simulink model "ElectricVehicle"  (R2022b)
settings: Solver=VariableStepAuto  StartTime=0  StopTime=350  RelTol=1e-3
libraries: autolibshared x1, slpidlib x1
settings Model: Creator=frz  LastModifiedBy=frz
settings SolverCC: ZeroCrossAlgorithm=Adaptive
settings DataIOCC: SaveOutput=off  SaveTime=off  ReturnWorkspaceOutputs=off
settings DebuggingCC: MaskedZcDiagnostic=none  IgnoredZcDiagnostic=none

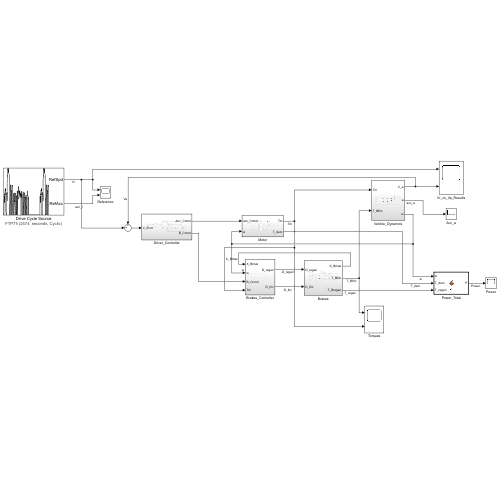
[thumbnail: Simulink's stored preview of the top-level diagram]
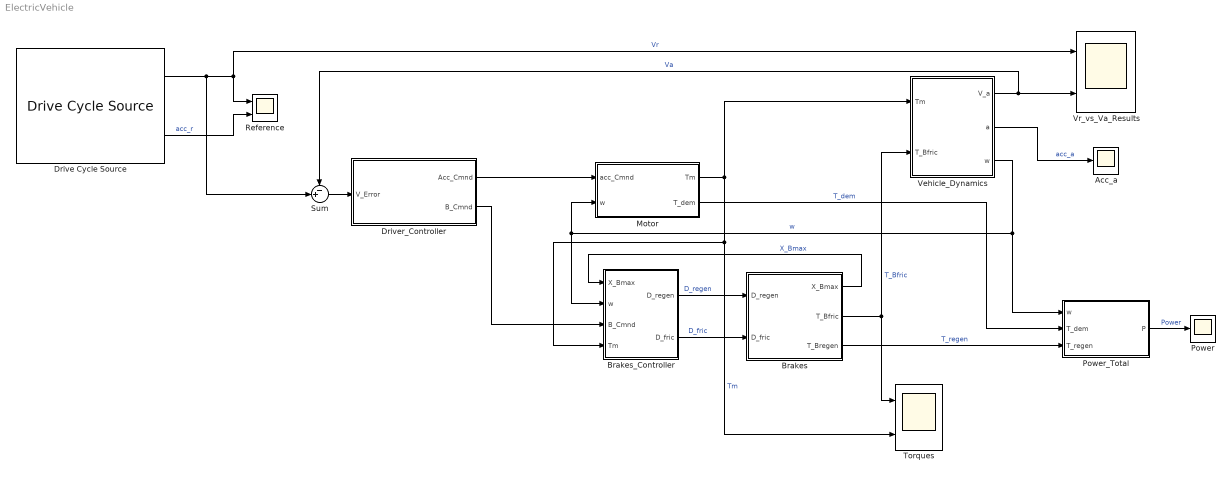
== system ElectricVehicle ==
  Acc_a : Scope
  Brakes : Subsystem
  Brakes_Controller : Subsystem
  Drive Cycle Source : autolibshared/Drive Cycle Source  cycleVar=FTP75  fileVar=cycleFTP75.mat  tfinal="2474  seconds, Cyclic"  cycleRepeat=on  outAccPort=on  outGearPort=off  gearList=No gear data  t_wot1=5  xdot_woto=0  xdot_wot1=30  t_wot2=20  xdot_wot2=0  t_wotend=30  srcUnit=m/s  outUnit=km/h  srcAccUnit=m/s/s  outAccUnit=m/s^2  dt=0  aMode=1  faultOption=off  velBnd=2  velBndUnit=mph  inUnit=m/s  timeBnd=1  failOption=off  stopSim=off  maxFaultCnt=10  maxFaultTime=2  maxTotFaultTime=15  traceOption=off  dtTrace=1  traceWindow=10  lastDCname=FTP75  lastOutUnit=mph  lastDT=0  lastTB=1  lastSB=2  forceCalcBound=off
  Driver_Controller : Subsystem
  Motor : Subsystem
  Power : Scope
  Power_Total : MATLAB Function  TreatAsAtomicUnit=on
  Reference : Scope  NumInputPorts=2
  Sum : Sum  Inputs=-+|
  Torques : Scope  NumInputPorts=2
  Vehicle_Dynamics : Subsystem
  Vr_vs_Va_Results : Scope  NumInputPorts=2
  wires:
  Drive Cycle Source/1 -> Sum/2, Reference/1, Vr_vs_Va_Results/1  "Vr"
  Drive Cycle Source/2 -> Reference/2  "acc_r"
  Brakes/2(T_Bfric) -> Vehicle_Dynamics/2(T_Bfric), Torques/1  "T_Bfric"
  Brakes/1(X_Bmax) -> Brakes_Controller/1(X_Bmax)  "X_Bmax"
  Brakes_Controller/1(D_regen) -> Brakes/1(D_regen)  "D_regen"
  Brakes_Controller/2(D_fric) -> Brakes/2(D_fric)  "D_fric"
  Brakes/3(T_Bregen) -> Power_Total/3(T_regen)  "T_regen"
  Vehicle_Dynamics/3(w) -> Power_Total/1(w), Motor/2(w), Brakes_Controller/2(w)  "w"
  Vehicle_Dynamics/1(V_a) -> Vr_vs_Va_Results/2, Sum/1  "Va"
  Driver_Controller/1(Acc_Cmnd) -> Motor/1(acc_Cmnd)
  Driver_Controller/2(B_Cmnd) -> Brakes_Controller/3(B_Cmnd)
  Sum/1 -> Driver_Controller/1(V_Error)
  Motor/1(Tm) -> Torques/2, Brakes_Controller/4(Tm), Vehicle_Dynamics/1(Tm)  "Tm"
  Vehicle_Dynamics/2(a) -> Acc_a/1  "acc_a"
  Motor/2(T_dem) -> Power_Total/2(T_dem)  "T_dem"
  Power_Total/1(P) -> Power/1  "Power"

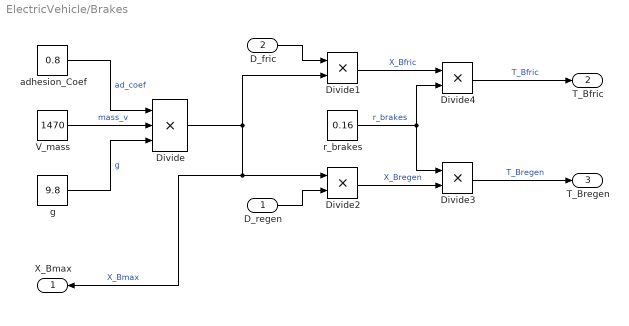
== system ElectricVehicle/Brakes ==
  D_regen : Inport
  D_fric : Inport  Port=2
  Divide : Product  Inputs=***
  Divide{1..4} (4 alike) : Product  Inputs=**
  V_mass : Constant  Value=1470
  adhesion_Coef : Constant  Value=0.8
  g : Constant  Value=9.8
  r_brakes : Constant  Value=0.16
  X_Bmax : Outport
  T_Bfric : Outport  Port=2
  T_Bregen : Outport  Port=3
  wires:
  g/1 -> Divide/3  "g"
  adhesion_Coef/1 -> Divide/1  "ad_coef"
  V_mass/1 -> Divide/2  "mass_v"
  D_fric/1 -> Divide1/1
  Divide1/1 -> Divide4/1  "X_Bfric"
  Divide4/1 -> T_Bfric/1  "T_Bfric"
  r_brakes/1 -> Divide3/1, Divide4/2  "r_brakes"
  D_regen/1 -> Divide2/2
  Divide/1 -> Divide1/2, X_Bmax/1, Divide2/1  "X_Bmax"
  Divide2/1 -> Divide3/2  "X_Bregen"
  Divide3/1 -> T_Bregen/1  "T_Bregen"

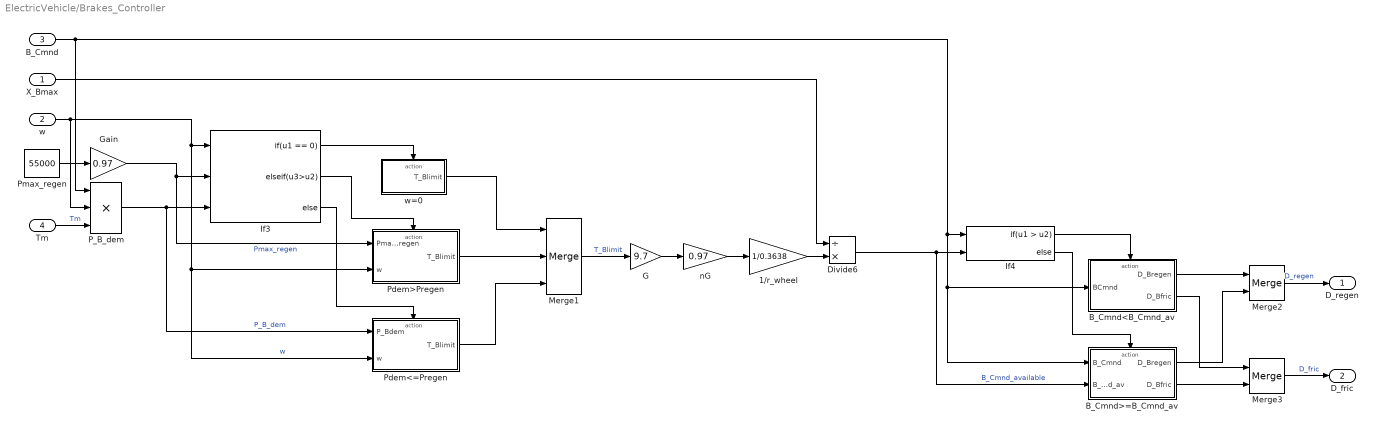
== system ElectricVehicle/Brakes_Controller ==
  X_Bmax : Inport
  w : Inport  Port=2
  B_Cmnd : Inport  Port=3
  Tm : Inport  Port=4
  1/r_wheel : Gain  Gain=1/0.3638
  B_Cmnd<B_Cmnd_av : Subsystem  TreatAsAtomicUnit=on
  B_Cmnd>=B_Cmnd_av : Subsystem  TreatAsAtomicUnit=on
  Divide6 : Product  Inputs=/*
  G : Gain  Gain=9.7
  Gain : Gain  Gain=0.97
  If3 : If  NumInputs=3  IfExpression=u1 == 0  ElseIfExpressions=u3>u2
  If4 : If  NumInputs=2  IfExpression=u1 > u2
  Merge1 : Merge  Inputs=3
  Merge2 : Merge
  Merge3 : Merge
  P_B_dem : Product  Inputs=***
  Pdem<=Pregen : Subsystem  TreatAsAtomicUnit=on
  Pdem>Pregen : Subsystem  TreatAsAtomicUnit=on
  Pmax_regen : Constant  Value=55000
  nG : Gain  Gain=0.97
  w=0 : Subsystem  TreatAsAtomicUnit=on
  D_regen : Outport
  D_fric : Outport  Port=2
  wires:
  Pdem<=Pregen/1(T_Blimit) -> Merge1/3
  If3/1 -> w=0/Action
  Pmax_regen/1 -> Gain/1
  B_Cmnd/1 -> If4/1, B_Cmnd<B_Cmnd_av/1(BCmnd), B_Cmnd>=B_Cmnd_av/1(B_Cmnd), P_B_dem/1
  X_Bmax/1 -> Divide6/1
  Merge2/1 -> D_regen/1  "D_regen"
  If3/2 -> Pdem>Pregen/Action
  P_B_dem/1 -> If3/3, Pdem<=Pregen/1(P_Bdem)  "P_B_dem"
  G/1 -> nG/1
  w/1 -> P_B_dem/2, Pdem>Pregen/2(w), Pdem<=Pregen/2(w), If3/1  "w"
  w=0/1(T_Blimit) -> Merge1/1
  Pdem>Pregen/1(T_Blimit) -> Merge1/2
  B_Cmnd>=B_Cmnd_av/2(D_Bfric) -> Merge3/2
  If3/3 -> Pdem<=Pregen/Action
  1/r_wheel/1 -> Divide6/2
  B_Cmnd<B_Cmnd_av/2(D_Bfric) -> Merge3/1
  B_Cmnd>=B_Cmnd_av/1(D_Bregen) -> Merge2/2
  If4/2 -> B_Cmnd>=B_Cmnd_av/Action
  Divide6/1 -> If4/2, B_Cmnd>=B_Cmnd_av/2(B_Cmnd_av)  "B_Cmnd_available"
  If4/1 -> B_Cmnd<B_Cmnd_av/Action
  nG/1 -> 1/r_wheel/1
  Merge1/1 -> G/1  "T_Blimit"
  B_Cmnd<B_Cmnd_av/1(D_Bregen) -> Merge2/1
  Merge3/1 -> D_fric/1  "D_fric"
  Gain/1 -> If3/2, Pdem>Pregen/1(Pmax_regen)  "Pmax_regen"
  Tm/1 -> P_B_dem/3  "Tm"

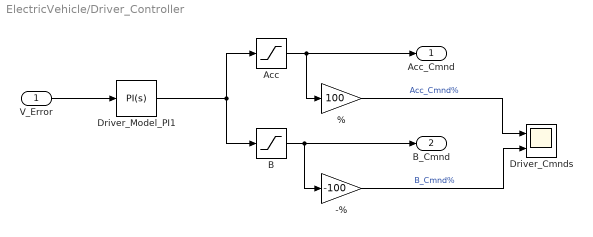
== system ElectricVehicle/Driver_Controller ==
  V_Error : Inport
  % : Gain  Gain=100
  -% : Gain  Gain=-100
  Acc : Saturate  UpperLimit=1  LowerLimit=0
  B : Saturate  UpperLimit=0  LowerLimit=-1
  Driver_Cmnds : Scope  NumInputPorts=2
  Driver_Model_PI1 : slpidlib/PID Controller  Controller=PI  Form=Parallel  TimeDomain=Continuous-time  UseExternalTs=off  SampleTime=-1  IntegratorMethod=Forward Euler  FilterMethod=Forward Euler  ControllerParametersSource=internal  P=1  I=0.01  UseKiTs=off  D=0  N=100  UseFilter=on  TunerSelectOption=Transfer Function Based (PID Tuner App)  InitialConditionSource=internal  InitialConditionForIntegrator=0  InitialConditionForFilter=0  DifferentiatorICPrevScaledInput=0  ExternalReset=none  TrackingMode=off  Kt=1  LimitOutput=off  SatLimitsSource=internal  UpperSaturationLimit=inf  LowerSaturationLimit=-inf  LinearizeAsGain=on  AntiWindupMode=none  Kb=1  LimitIntegrator=off  UpperIntegratorSaturationLimit=inf  LowerIntegratorSaturationLimit=-inf  POutMin=[]  POutMax=[]  IOutMin=[]  IOutMax=[]  DOutMin=[]  DOutMax=[]  NOutMin=[]  NOutMax=[]  SumOutMin=[]  SumOutMax=[]  SaturationOutMin=[]  SaturationOutMax=[]  PParamMin=[]  PParamMax=[]  IParamMin=[]  IParamMax=[]  DParamMin=[]  DParamMax=[]  NParamMin=[]  NParamMax=[]  KbParamMin=[]  KbParamMax=[]  KtParamMin=[]  KtParamMax=[]  KbOutMin=[]  KbOutMax=[]  KtOutMin=[]  KtOutMax=[]  IntegratorOutMin=[]  IntegratorOutMax=[]  FilterOutMin=[]  FilterOutMax=[]  SumI1OutMin=[]  SumI1OutMax=[]  SumI2OutMin=[]  SumI2OutMax=[]  SumI3OutMin=[]  SumI3OutMax=[]  SumI4OutMin=[]  SumI4OutMax=[]  SumDOutMin=[]  SumDOutMax=[]  DifferentiatorOutMin=[]  DifferentiatorOutMax=[]  FilterDiffOutCoefMin=[]  FilterDiffOutCoefMax=[]  ReciprocalOutMin=[]  ReciprocalOutMax=[]  SumDenOutMin=[]  SumDenOutMax=[]  SumNumOutMin=[]  SumNumOutMax=[]  DivideOutMin=[]  DivideOutMax=[]  UdiffTsProdOutMin=[]  UdiffTsProdOutMax=[]  NTsProdOutMin=[]  NTsProdOutMax=[]  UintegralTsProdOutMin=[]  UintegralTsProdOutMax=[]  UngainTsProdOutMin=[]  UngainTsProdOutMax=[]  ClampingZeroOutDataTypeStr=Inherit: Inherit via back propagation  ClampingZeroOutMin=[]  ClampingZeroOutMax=[]  FilterDenConstantOutDataTypeStr=Inherit: Inherit via back propagation  FilterDenConstantOutMin=[]  FilterDenConstantOutMax=[]  PCopyOutDataTypeStr=Inherit: Inherit via back propagation  PCopyOutMin=[]  PCopyOutMax=[]  NCopyOutDataTypeStr=Inherit: Inherit via back propagation  NCopyOutMin=[]  NCopyOutMax=[]  IntegratorContinuousStateAttributes=''  IntegratorStateMustResolveToSignalObject=off  IntegratorRTWStateStorageClass=Auto  FilterContinuousStateAttributes=''  FilterStateMustResolveToSignalObject=off  FilterRTWStateStorageClass=Auto  ParallelPVariant=InternalParameters  IdealPVariant=Disabled  IVariant=InternalParameters  DVariant=Disabled  IntegratorVariant=Continuous  SatVariant=Disabled  AWVariant=Passthrough  PCopyVariant=Disabled  TRVariant=Disabled  FdbkBlocksVariant=Forward  IdealPFdbkVariant=Disabled  SatFdbkVariant=Disabled  DerivativeFilterVariant=Disabled  NVariant=Disabled  NCopyVariant=Disabled_SignalSpec  FilterICVariant=Disabled  IntegratorICVariant=InternalICs  ExternalResetVariant=Disabled  TRSumVariant=Passthrough  SumFdbkVariant=Disabled  SumVariant=Sum_PI  TsampFilterVariant=InternalTs  TsampNgainVariant=Passthrough  TsampIntegralVariant=Passthrough  ExternalSaturationOutDataTypeStr=Inherit: Same as second input
  Acc_Cmnd : Outport
  B_Cmnd : Outport  Port=2
  wires:
  Driver_Model_PI1/1 -> Acc/1, B/1
  %/1 -> Driver_Cmnds/1  "Acc_Cmnd%"
  B/1 -> B_Cmnd/1, -%/1
  Acc/1 -> Acc_Cmnd/1, %/1
  V_Error/1 -> Driver_Model_PI1/1
  -%/1 -> Driver_Cmnds/2  "B_Cmnd%"

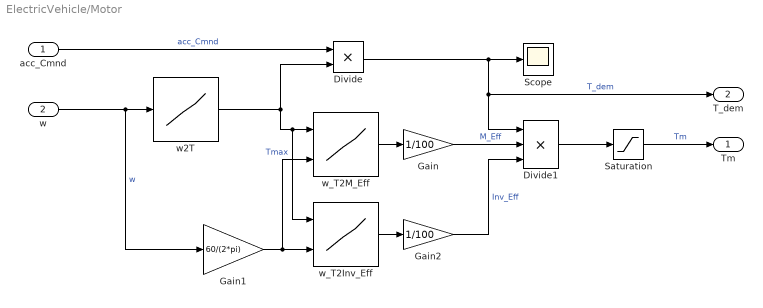
== system ElectricVehicle/Motor ==
  acc_Cmnd : Inport
  w : Inport  Port=2
  Divide : Product  Inputs=**
  Divide1 : Product  Inputs=***
  Gain : Gain  Gain=1/100
  Gain1 : Gain  Gain=60/(2*pi)
  Gain2 : Gain  Gain=1/100
  Saturation : Saturate  UpperLimit=250  LowerLimit=-250
  Scope : Scope
  w2T : Lookup_n-D  NumberOfTableDimensions=1  BreakpointsForDimension1=[0;4700;11400]  Table=[250;250;89]  InternalRulePriority=Speed  RndMeth=Simplest
  w_T2Inv_Eff : Lookup_n-D  BreakpointsForDimension1=[0;50;100;150;200;250]  BreakpointsForDimension2=[0;1000;1200;1400;1600;1800;2000;2300;3000;4000;5000;6000;7000;8000;9000;10000;12000]  Table=[84 86 88 90 91 92 93 94 95 96 97 98 98 98 98 98 98;84 86 88 90 91 92 93 94 96 97 97 98 98 99 99 98 99;86 88 90 91 92 93 94 95 96 97 98 98 99 99 99 99 99;86 88 90 91 92 93 94 95 96 97 98 98 98 99 0 0 0;86 88 90 91 92 93 94 95 96 97 98 98 0 0 0 0 0;86 88 90 91 92 93 94 95 96 97 0 0 0 0 0 0 0]  InternalRulePriority=Speed  RndMeth=Simplest
      settings: InputPortMap=u0,u1
  w_T2M_Eff : Lookup_n-D  BreakpointsForDimension1=[0;100;200;250]  BreakpointsForDimension2=[0;30;50;70;100;500;700;4000;5000;12000]  Table=[60 70 80 85 90 95 97 60 60 90;60 70 80 85 90 95 95 97 97 95;70 80 85 85 90 95 95 97 97 0;70 80 85 80 85 90 95 95 97 0]  InternalRulePriority=Speed  RndMeth=Simplest
      settings: InputPortMap=u0,u1
  Tm : Outport
  T_dem : Outport  Port=2
  wires:
  w2T/1 -> w_T2Inv_Eff/1, w_T2M_Eff/1, Divide/2  "Tmax"
  w/1 -> Gain1/1, w2T/1  "w"
  Divide/1 -> Scope/1, Divide1/1, T_dem/1  "T_dem"
  Saturation/1 -> Tm/1  "Tm"
  acc_Cmnd/1 -> Divide/1  "acc_Cmnd"
  Divide1/1 -> Saturation/1
  Gain/1 -> Divide1/2  "M_Eff"
  Gain1/1 -> w_T2Inv_Eff/2, w_T2M_Eff/2
  w_T2M_Eff/1 -> Gain/1
  w_T2Inv_Eff/1 -> Gain2/1
  Gain2/1 -> Divide1/3  "Inv_Eff"

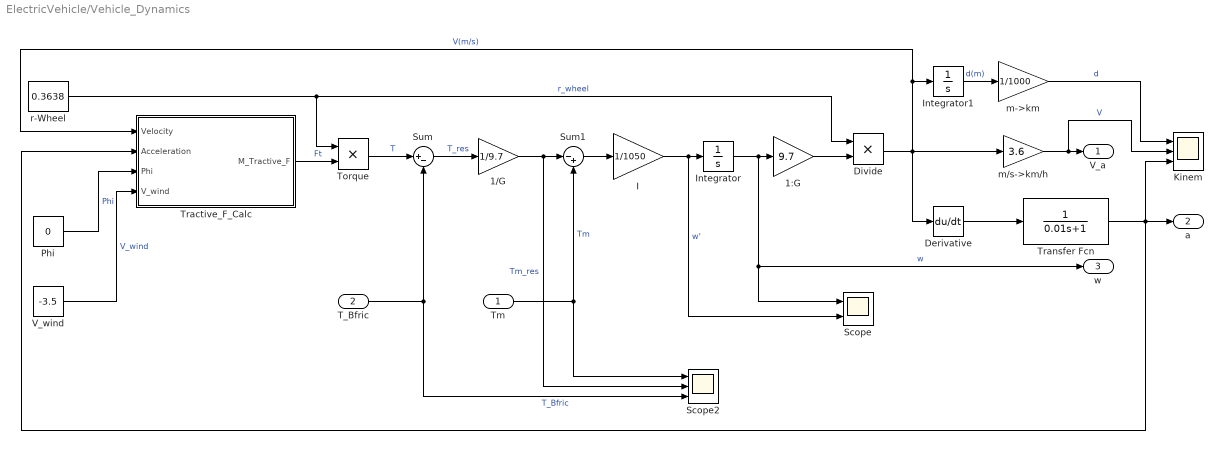
== system ElectricVehicle/Vehicle_Dynamics ==
  Tm : Inport
  T_Bfric : Inport  Port=2
  1/G : Gain  Gain=1/9.7
  1:G : Gain  Gain=9.7
  Derivative : Derivative
  Divide : Product  Inputs=**
  I : Gain  Gain=1/1050
  Integrator : Integrator  LimitOutput=on  UpperSaturationLimit=11400*2*pi/60  LowerSaturationLimit=-11400*2*pi/60
  Integrator1 : Integrator
  Kinem : Scope  NumInputPorts=3
  Phi : Constant  Value=0
  Scope : Scope  NumInputPorts=2
  Scope2 : Scope  NumInputPorts=3
  Sum : Sum  Inputs=|+-
  Sum1 : Sum  Inputs=|-+
  Torque : Product  Inputs=**
  Tractive_F_Calc : Subsystem
  Transfer Fcn : TransferFcn  Denominator=[0.01 1]
  V_wind : Constant  Value=-3.5
  m->km : Gain  Gain=1/1000
  m/s->km/h : Gain  Gain=3.6
  r-Wheel : Constant  Value=0.3638
  V_a : Outport
  a : Outport  Port=2
  w : Outport  Port=3
  wires:
  m->km/1 -> Kinem/1  "d"
  Sum1/1 -> I/1
  Divide/1 -> Tractive_F_Calc/1(Velocity), Integrator1/1, m/s->km/h/1, Derivative/1  "V(m/s)"
  1:G/1 -> Divide/2
  r-Wheel/1 -> Divide/1, Torque/1  "r_wheel"
  Integrator1/1 -> m->km/1  "d(m)"
  Torque/1 -> Sum/1  "T"
  Integrator/1 -> Scope/1, w/1, 1:G/1  "w"
  Sum/1 -> 1/G/1  "T_res"
  V_wind/1 -> Tractive_F_Calc/4(V_wind)  "V_wind"
  I/1 -> Scope/2, Integrator/1  "w'"
  T_Bfric/1 -> Scope2/3, Sum/2  "T_Bfric"
  Tractive_F_Calc/1(M_Tractive_F) -> Torque/2  "Ft"
  Phi/1 -> Tractive_F_Calc/3(Phi)  "Phi"
  Tm/1 -> Scope2/1, Sum1/2  "Tm"
  1/G/1 -> Scope2/2, Sum1/1  "Tm_res"
  m/s->km/h/1 -> Kinem/2, V_a/1  "V"
  Derivative/1 -> Transfer Fcn/1
  Transfer Fcn/1 -> a/1, Tractive_F_Calc/2(Acceleration), Kinem/3

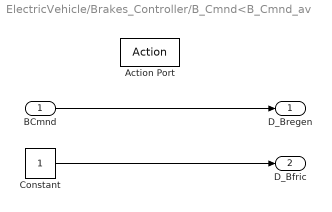
== system ElectricVehicle/Brakes_Controller/B_Cmnd<B_Cmnd_av ==
  BCmnd : Inport
  Action Port : ActionPort  ActionPortLabel=if(u1 > u2)
  Constant : Constant
  D_Bregen : Outport
  D_Bfric : Outport  Port=2
  wires:
  BCmnd/1 -> D_Bregen/1
  Constant/1 -> D_Bfric/1

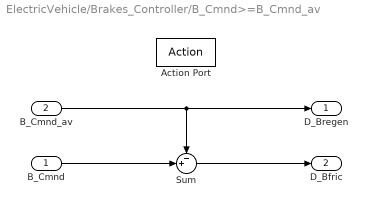
== system ElectricVehicle/Brakes_Controller/B_Cmnd>=B_Cmnd_av ==
  B_Cmnd : Inport
  B_Cmnd_av : Inport  Port=2
  Action Port : ActionPort  ActionPortLabel=else
  Sum : Sum  Inputs=-+|
  D_Bregen : Outport
  D_Bfric : Outport  Port=2
  wires:
  B_Cmnd_av/1 -> Sum/1, D_Bregen/1
  B_Cmnd/1 -> Sum/2
  Sum/1 -> D_Bfric/1

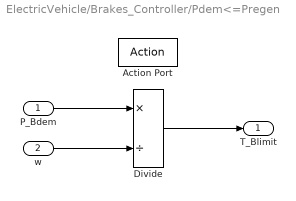
== system ElectricVehicle/Brakes_Controller/Pdem<=Pregen ==
  P_Bdem : Inport
  w : Inport  Port=2
  Action Port : ActionPort  ActionPortLabel=else
  Divide : Product  Inputs=*/
  T_Blimit : Outport
  wires:
  P_Bdem/1 -> Divide/1
  w/1 -> Divide/2
  Divide/1 -> T_Blimit/1

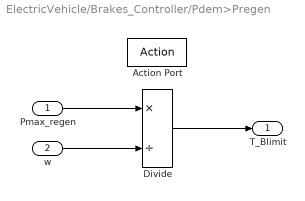
== system ElectricVehicle/Brakes_Controller/Pdem>Pregen ==
  Pmax_regen : Inport
  w : Inport  Port=2
  Action Port : ActionPort  ActionPortLabel=elseif(u3>u2)
  Divide : Product  Inputs=*/
  T_Blimit : Outport
  wires:
  Pmax_regen/1 -> Divide/1
  w/1 -> Divide/2
  Divide/1 -> T_Blimit/1

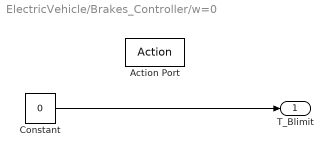
== system ElectricVehicle/Brakes_Controller/w=0 ==
  Action Port : ActionPort  ActionPortLabel=if(u1 == 0)
  Constant : Constant  Value=0
  T_Blimit : Outport
  wires:
  Constant/1 -> T_Blimit/1

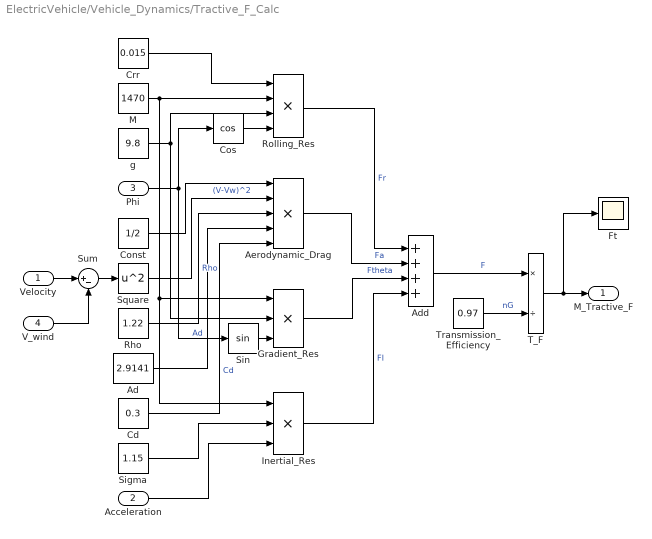
== system ElectricVehicle/Vehicle_Dynamics/Tractive_F_Calc ==
  Velocity : Inport
  Acceleration : Inport  Port=2
  Phi : Inport  Port=3
  V_wind : Inport  Port=4
  Ad : Constant  Value=2.9141
  Add : Sum  Inputs=++++
  Aerodynamic_Drag : Product  Inputs=*****
  Cd : Constant  Value=0.3
  Const : Constant  Value=1/2
  Cos : Trigonometry  Operator=cos
  Crr : Constant  Value=0.015
  Ft : Scope
  Gradient_Res : Product  Inputs=***
  Inertial_Res : Product  Inputs=***
  M : Constant  Value=1470
  Rho : Constant  Value=1.22
  Rolling_Res : Product  Inputs=****
  Sigma : Constant  Value=1.15
  Sin : Trigonometry
  Square : Math  Operator=square
  Sum : Sum  Inputs=|+-
  T_F : Product  Inputs=*/
  Transmission_Efficiency : Constant  Value=0.97
  g : Constant  Value=9.8
  M_Tractive_F : Outport
  wires:
  Rolling_Res/1 -> Add/1  "Fr"
  Sin/1 -> Gradient_Res/3
  Cd/1 -> Aerodynamic_Drag/5  "Cd"
  Add/1 -> T_F/1  "F"
  Inertial_Res/1 -> Add/4  "FI"
  Aerodynamic_Drag/1 -> Add/2  "Fa"
  M/1 -> Inertial_Res/1, Gradient_Res/1, Rolling_Res/2
  Crr/1 -> Rolling_Res/1
  Sigma/1 -> Inertial_Res/2
  Acceleration/1 -> Inertial_Res/3
  g/1 -> Gradient_Res/2, Rolling_Res/3
  Cos/1 -> Rolling_Res/4
  Sum/1 -> Square/1
  Gradient_Res/1 -> Add/3  "Ftheta"
  T_F/1 -> Ft/1, M_Tractive_F/1
  Velocity/1 -> Sum/1
  Ad/1 -> Aerodynamic_Drag/4  "Ad"
  Rho/1 -> Aerodynamic_Drag/3  "Rho"
  Const/1 -> Aerodynamic_Drag/1
  Transmission_Efficiency/1 -> T_F/2  "nG"
  Square/1 -> Aerodynamic_Drag/2  "(V-Vw)^2"
  Phi/1 -> Cos/1, Sin/1
  V_wind/1 -> Sum/2

== matlab function ElectricVehicle/Power_Total ==
  data: w input; T_dem input; P output; T_regen input
function P = fcn(w,T_dem, T_regen)
T = T_dem - T_regen;
P_driv = T*w;

ACond = 500;
Aud = 35;
DrCtrl = 150;
EMS = 150;
MLights = 120;
SLamps = 50;
Horn = 10;
Steering = 400;
W = 80;
WDef = 250;
Wip = 40;
P_ac = ACond+Aud+DrCtrl+EMS+MLights+SLamps+Horn+Steering+W+WDef+Wip;

B_eff = 0.95;
Conv_eff = 0.9;
P_aux = P_ac*B_eff*Conv_eff;

Power = P_driv + P_aux;

P = Power;
